simulink model "kalman_simulink"  (R2019b)
settings: Solver=VariableStepAuto  StartTime=0.0  StopTime=10.0  RelTol=1e-3
libraries: simulink x2, shared6dof x1
settings Model: Creator=Lightning  LastModifiedBy=Lightning

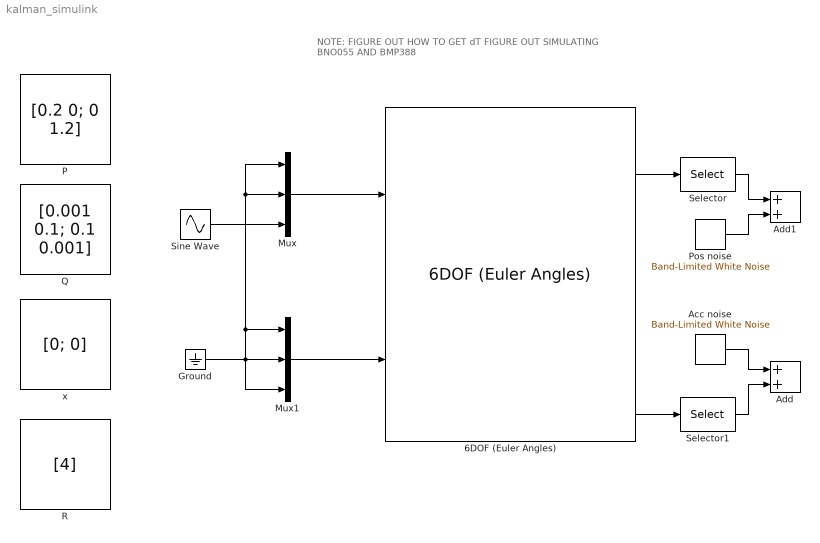
== system kalman_simulink ==
  note: NOTE:
      | FIGURE OUT HOW TO GET dT
      | FIGURE OUT SIMULATING BNO055 AND BMP388
  6DOF (Euler Angles) : shared6dof/6DOF (Euler Angles)  units=Metric (MKS)  mtype=Fixed  rep=Euler Angles  xme_0=[0 0 0]  Vm_0=[0 0 0]  eul_0=[0 0 0]  pm_0=[0 0 0]  mass_0=1.0  mass_e=0.5  mass_f=2.0  inertia=eye(3)  inertia_e=eye(3)  inertia_f=2*eye(3)  k_quat=1.0  vre_flag=on  abi_flag=off  aMode=0  xme_statename=''  Vm_statename=''  eul_statename=''  quat_statename=''  pm_statename=''  mass_statename=''
      settings: SourceProductBaseCode=AE
  Acc noise : simulink/Sources/Band-Limited White Noise  Cov=0.008  Ts=0.1  seed=[23341]
  Add : Sum
  Add1 : Sum
  Ground : Ground
  Mux : Mux  Inputs=3
  Mux1 : Mux  Inputs=3
  P : Constant  Value=[0.2 0; 0 1.2]  VectorParams1D=off
  Pos noise : simulink/Sources/Band-Limited White Noise  Cov=0.01  Ts=0.1  seed=[23341]
  Q : Constant  Value=[0.001 0.1; 0.1 0.001]  VectorParams1D=off
  R : Constant  Value=[4]  VectorParams1D=off
  Selector : Selector  InputPortWidth=3  IndexOptions=Index vector (dialog)  Indices=[3]  OutputSizes=1
  Selector1 : Selector  InputPortWidth=3  IndexOptions=Index vector (dialog)  Indices=[3]  OutputSizes=1
  Sine Wave : Sin  Amplitude=5  Bias=5  SampleTime=0
  x : Constant  Value=[0; 0]  VectorParams1D=off
  wires:
  Mux/1 -> 6DOF (Euler Angles)/1
  Ground/1 -> Mux1/3, Mux1/2, Mux1/1, Mux/1, Mux/2
  Mux1/1 -> 6DOF (Euler Angles)/2
  Sine Wave/1 -> Mux/3
  6DOF (Euler Angles)/2 -> Selector/1
  6DOF (Euler Angles)/8 -> Selector1/1
  Selector1/1 -> Add/2
  Acc noise/1 -> Add/1
  Pos noise/1 -> Add1/2
  Selector/1 -> Add1/1
